simulink model "Simulink_PMSM"  (R2022b)
settings: Solver=VariableStepAuto  StartTime=0.0  StopTime=3.5  FixedStep=Ts  MaxStep=1e-5  RelTol=1e-3  AbsTol=1e-3  EnableMultiTasking=on
PreLoadFcn:
  | % PMSM parameters
  | PM = 0.005237624506507; % Permanent magnet flux linkage
  | Ld = 0.00105;  % d-axis inductance
  | Lq = 0.00105;  % q-axis inductance
  | L0 = 0.00105;  % 0-axis inductance
  | Rs = 0.75; % Stator resistance
  | N = 4; % Number of pole pairs
  | J = 2.4018552467e-06; % Moment of inertia
  | B = 1.160371049300000e-05; % Damping
  | 
  | % Operating and derived limits
  | Trated = 0.056566344670276 %Par nominal
values from neighbouring files (symbols this model uses):
  fsw = 1e3    (= 1000)    [Variables_simulink_PMSM.m]
  Kiid = 2    [Variables_simulink_PMSM.m]
  Kiiq = Kpiq    (= 1)    [Variables_simulink_PMSM.m]
  Kivel = 3    [Variables_simulink_PMSM.m]
  Kpid = 1    [Variables_simulink_PMSM.m]
  Kpiq = Kpid    (= 1)    [Variables_simulink_PMSM.m]
  Kpvel = 6    [Variables_simulink_PMSM.m]
  Refvel = 300    [Variables_simulink_PMSM.m]
  Tcurr = 1e-4    (= 0.0001)    [Variables_simulink_PMSM.m]
  Ts = 1e-6    (= 1e-06)    [Variables_simulink_PMSM.m]
  Tspeed = 2e-4    (= 0.0002)    [Variables_simulink_PMSM.m]
  Tsw = 5e-7    (= 5e-07)    [Variables_simulink_PMSM.m]
  Vbat = 48    [Variables_simulink_PMSM.m]
libraries: slpidlib x3, eePwmGenerator x3, eeTransforms x2, simulink x1, eePwmGeneratorTwoLevel x1, autolibpmsmexterior x1
Description:
  | Three-Phase PMSM Drive
settings Model: Creator=The MathWorks, Inc.  LastModifiedBy=emate
settings SolverCC: AutoScaleAbsTol=off  MaxConsecutiveMinStep=2  ZeroCrossAlgorithm=Adaptive  AlgebraicLoopSolver=TrustRegion  MaxZcPerStep=1
settings DataIOCC: LimitDataPoints=on  MaxDataPoints=690000  SaveFormat=Array  ReturnWorkspaceOutputs=off  SignalLoggingName=logsout_ee_pmsm_drive
settings OptimizationCC: LifeSpan=inf
settings DebuggingCC: MaxConsecutiveZCsMsg=none  IgnoredZcDiagnostic=none  UnconnectedInputMsg=warning  UnconnectedOutputMsg=warning  UnconnectedLineMsg=warning  AllowSymbolicDim=off  PregeneratedLibrarySubsystemCodeDiagnostic=none  SFUnexpectedBacktrackingDiag=warning  SFNoUnconditionalDefaultTransitionDiag=warning  SFExecutionAtInitializationDiag=none  SFMachineParentedDataDiag=warning  ArithmeticOperatorsInVariantConditions=warning
settings HardwareCC: ProdBitPerPointer=32  ProdBitPerSizeT=32  ProdBitPerPtrDiffT=32  ProdLargestAtomicFloat=None  ProdIntDivRoundTo=Undefined  ProdEndianess=Unspecified  ProdWordSize=32  ProdHWDeviceType=32-bit Generic
settings ModelReferenceCC: EnableRefExpFcnMdlSchedulingChecks=on  PropagateSignalLabelsOutOfModel=off
settings SFSimCC: SimUseLocalCustomCode=off
settings RTWCC: RTWUseLocalCustomCode=off  DLArmComputeVersion=19.05
settings CodeAppCC: StateflowObjectComments=on
settings GRTTargetCC: TargetLangStandard=C89/C90 (ANSI)
settings ConfigComp: CovMetricSettings=dw  CovSaveCumulativeToWorkspaceVar=on  CovSaveSingleToWorkspaceVar=on  CovExternalEMLEnable=off  CovSFcnEnable=off
settings SimscapeCC: SimscapeLogType=all  SimscapeLogSimulationStatistics=on  SimscapeLogName=simlog_ee_pmsm_drive  SimscapeLogDataHistory=690000

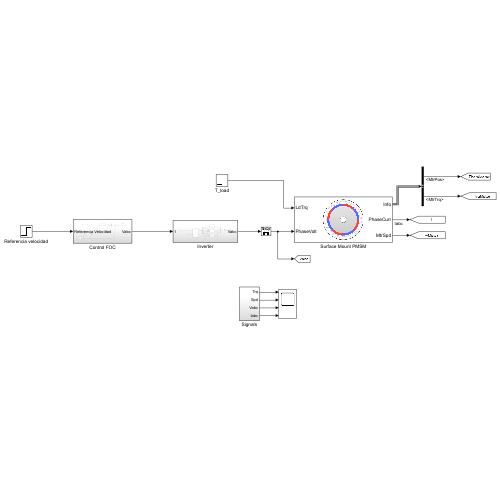
[thumbnail: Simulink's stored preview of the top-level diagram]
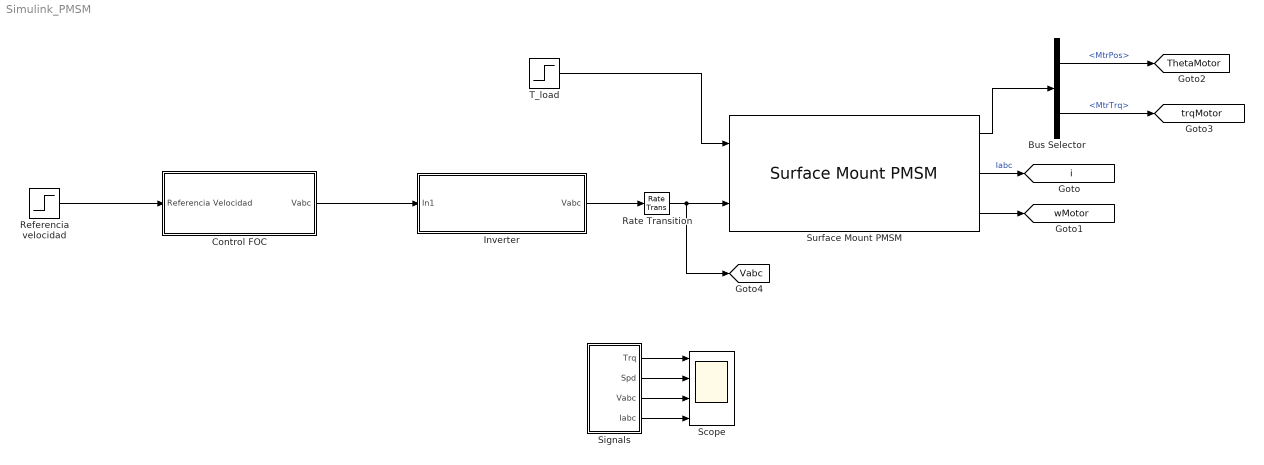
== system Simulink_PMSM ==
  Bus Selector : BusSelector  OutputSignals=MtrPos,MtrTrq
  Control FOC : Subsystem
  Inverter : Subsystem
  Rate Transition : RateTransition  Deterministic=off  OutPortSampleTime=Tsw
  Referencia velocidad : Step  Time=0.5  After=Refvel  SampleTime=Tspeed
  Scope : Scope  NumInputPorts=4
  "Signals " : Subsystem
  Surface Mount PMSM : autolibpmsmexterior/Surface Mount PMSM  port_config=Torque  sim_type=Discrete  Ts=Ts  P=N  Rs=Rs  Ldq_=Ld  KConstText=Permanent flux linkage constant (lambda_pm):  lambda_pm=PM  Ke=159.9771  Kt=1.323  mechanical=[J*1e4, B*5, 0]  idq0=[0 0]  theta_init=0  omega_init=0  KConst=PM  lambda_pm_calc=PM  RefBlkName='autolibpmsmexterior/Surface Mount PMSM'  aMode=5  Ldq="[0.0006      0.0006]"
  T_load : Step  Time=2  After=0.75*Trated  SampleTime=Ts
  tag scope: ThetaMotor=global, Vabc=global, i=global, trqMotor=global, wMotor=global
  wires:
  "Signals "/2(Spd) -> Scope/2
  "Signals "/1(Trq) -> Scope/1
  "Signals "/3(Vabc) -> Scope/3
  "Signals "/4(Iabc) -> Scope/4
  Referencia velocidad/1 -> Control FOC/1(Referencia Velocidad)
  Control FOC/1(Vabc) -> Inverter/1(In1)
  Rate Transition/1 -> [Vabc], Surface Mount PMSM/2
  T_load/1 -> Surface Mount PMSM/1
  Surface Mount PMSM/3 -> [wMotor]
  Surface Mount PMSM/2 -> [i]  "Iabc"
  Surface Mount PMSM/1 -> Bus Selector/1
  Bus Selector/1 -> [ThetaMotor]  "<MtrPos>"
  Bus Selector/2 -> [trqMotor]  "<MtrTrq>"
  Inverter/1(Vabc) -> Rate Transition/1

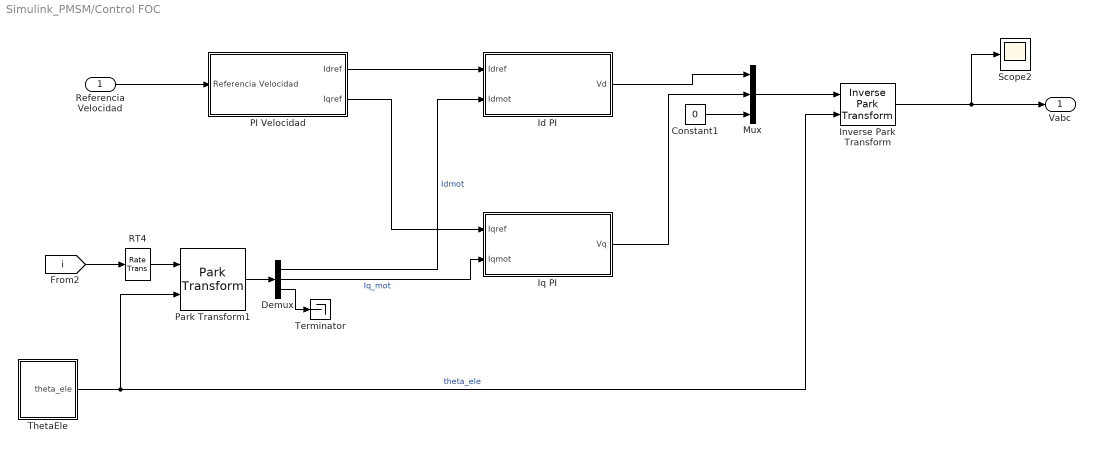
== system Simulink_PMSM/Control FOC ==
  Referencia Velocidad : Inport
  Constant1 : Constant  Value=0  SampleTime=Tcurr
  Demux : Demux  Outputs=3
  Id PI : Subsystem
  Inverse Park Transform : eeTransforms/Inverse Park Transform  AxisAlignment=D-axis  PowerInvariant=off
  Iq PI : Subsystem
  Mux : Mux  Inputs=3
  PI Velocidad : Subsystem
  Park Transform1 : eeTransforms/Park Transform  AxisAlignment=D-axis  PowerInvariant=off
      settings: LibrarySourceBlock=|
      | ee_sl_lib/Mathematical
      | Transforms/Park Transform
  RT4 : RateTransition  InitialCondition=[0,0,0]  OutPortSampleTime=Tspeed
  Scope2 : Scope
  Terminator : Terminator
  ThetaEle : Subsystem
  Vabc : Outport
  wires:
  PI Velocidad/1(Idref) -> Id PI/1(Idref)
  Constant1/1 -> Mux/3
  PI Velocidad/2(Iqref) -> Iq PI/1(Iqref)
  [i] -> RT4/1
  Demux/2 -> Iq PI/2(Iqmot)  "Iq_mot"
  ThetaEle/1(theta_ele) -> Inverse Park Transform/2, Park Transform1/2  "theta_ele"
  Iq PI/1(Vq) -> Mux/2
  Id PI/1(Vd) -> Mux/1
  Inverse Park Transform/1 -> Scope2/1, Vabc/1
  Demux/3 -> Terminator/1
  Demux/1 -> Id PI/2(Idmot)  "Idmot"
  Park Transform1/1 -> Demux/1
  RT4/1 -> Park Transform1/1
  Mux/1 -> Inverse Park Transform/1
  Referencia Velocidad/1 -> PI Velocidad/1(Referencia Velocidad)

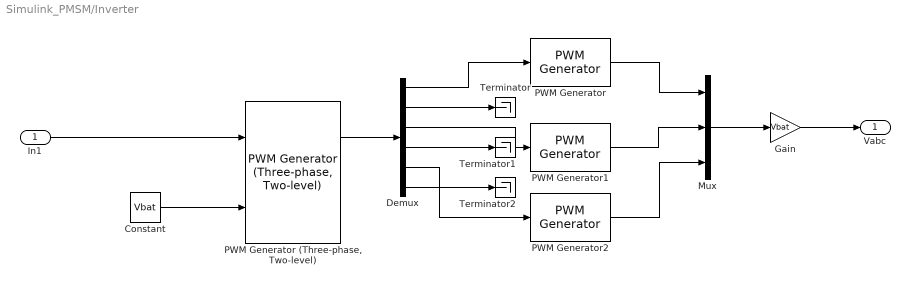
== system Simulink_PMSM/Inverter ==
  In1 : Inport
  Constant : Constant  Value=Vbat
  Demux : Demux  Outputs=6
  Gain : Gain  Gain=Vbat
  Mux : Mux  Inputs=3
  PWM Generator : eePwmGenerator/PWM Generator  CarrCount=Up  Tper=1/fsw  Tdelay=0  Ts=Tsw
  "PWM Generator (Three-phase, Two-level)" : eePwmGeneratorTwoLevel/PWM Generator (Three-phase, Two-level)  PWMMode=Continuous PWM (CPWM)  CPWMMode=SPWM: sinusoidal PWM  DPWMMode=60 DPWM: 60 degree discontinuous PWM  fsw=fsw  Ts=Tsw
      settings: LibrarySourceBlock=|
      | eePmsmFieldOrientedControl/PMSM Field-Oriented
      | Control/PWM/PWM Generator
      | (Three-phase, Two-level)
  PWM Generator1 : eePwmGenerator/PWM Generator  CarrCount=Up  Tper=1/fsw  Tdelay=0  Ts=Tsw
  PWM Generator2 : eePwmGenerator/PWM Generator  CarrCount=Up  Tper=1/fsw  Tdelay=0  Ts=Tsw
  Terminator : Terminator
  Terminator1 : Terminator
  Terminator2 : Terminator
  Vabc : Outport  VectorParamsAs1DForOutWhenUnconnected=off
  wires:
  In1/1 -> "PWM Generator (Three-phase, Two-level)"/1
  Mux/1 -> Gain/1
  Constant/1 -> "PWM Generator (Three-phase, Two-level)"/2
  "PWM Generator (Three-phase, Two-level)"/1 -> Demux/1
  Demux/2 -> Terminator/1
  Demux/4 -> Terminator1/1
  Demux/6 -> Terminator2/1
  PWM Generator/1 -> Mux/1
  Demux/1 -> PWM Generator/1
  Demux/3 -> PWM Generator1/1
  Demux/5 -> PWM Generator2/1
  PWM Generator1/1 -> Mux/2
  PWM Generator2/1 -> Mux/3
  Gain/1 -> Vabc/1

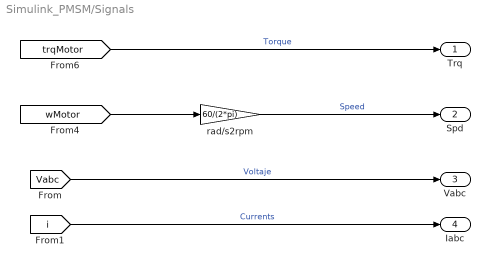
== system Simulink_PMSM/Signals  ==
  rad/s2rpm : Gain  Gain=60/(2*pi)
  Trq : Outport  VectorParamsAs1DForOutWhenUnconnected=off
  Spd : Outport  Port=2  VectorParamsAs1DForOutWhenUnconnected=off
  Vabc : Outport  Port=3  VectorParamsAs1DForOutWhenUnconnected=off
  Iabc : Outport  Port=4  VectorParamsAs1DForOutWhenUnconnected=off
  wires:
  [wMotor] -> rad/s2rpm/1
  [trqMotor] -> Trq/1  "Torque"
  [Vabc] -> Vabc/1  "Voltaje"
  rad/s2rpm/1 -> Spd/1  "Speed"
  [i] -> Iabc/1  "Currents"

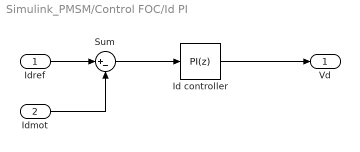
== system Simulink_PMSM/Control FOC/Id PI ==
  Idref : Inport
  Idmot : Inport  Port=2
  Id controller : slpidlib/PID Controller  Controller=PI  Form=Parallel  TimeDomain=Discrete-time  UseExternalTs=off  SampleTime=Tcurr  IntegratorMethod=Forward Euler  FilterMethod=Forward Euler  ControllerParametersSource=internal  P=Kpid  I=Kiid  UseKiTs=off  D=0  N=100  UseFilter=on  TunerSelectOption=Transfer Function Based (PID Tuner App)  InitialConditionSource=internal  InitialConditionForIntegrator=0  InitialConditionForFilter=0  DifferentiatorICPrevScaledInput=0  ExternalReset=none  TrackingMode=off  Kt=1  LimitOutput=on  SatLimitsSource=internal  UpperSaturationLimit=inf  LowerSaturationLimit=-inf  LinearizeAsGain=on  AntiWindupMode=clamping  Kb=1000  LimitIntegrator=off  UpperIntegratorSaturationLimit=inf  LowerIntegratorSaturationLimit=-inf  POutMin=[]  POutMax=[]  IOutMin=[]  IOutMax=[]  DOutMin=[]  DOutMax=[]  NOutMin=[]  NOutMax=[]  SumOutMin=[]  SumOutMax=[]  SaturationOutMin=[]  SaturationOutMax=[]  PParamMin=[]  PParamMax=[]  IParamMin=[]  IParamMax=[]  DParamMin=[]  DParamMax=[]  NParamMin=[]  NParamMax=[]  KbParamMin=[]  KbParamMax=[]  KtParamMin=[]  KtParamMax=[]  KbOutMin=[]  KbOutMax=[]  KtOutMin=[]  KtOutMax=[]  IntegratorOutMin=[]  IntegratorOutMax=[]  FilterOutMin=[]  FilterOutMax=[]  SumI1OutMin=[]  SumI1OutMax=[]  SumI2OutMin=[]  SumI2OutMax=[]  SumI3OutMin=[]  SumI3OutMax=[]  SumI4OutMin=[]  SumI4OutMax=[]  SumDOutMin=[]  SumDOutMax=[]  DifferentiatorOutMin=[]  DifferentiatorOutMax=[]  FilterDiffOutCoefMin=[]  FilterDiffOutCoefMax=[]  ReciprocalOutMin=[]  ReciprocalOutMax=[]  SumDenOutMin=[]  SumDenOutMax=[]  SumNumOutMin=[]  SumNumOutMax=[]  DivideOutMin=[]  DivideOutMax=[]  UdiffTsProdOutMin=[]  UdiffTsProdOutMax=[]  NTsProdOutMin=[]  NTsProdOutMax=[]  UintegralTsProdOutMin=[]  UintegralTsProdOutMax=[]  UngainTsProdOutMin=[]  UngainTsProdOutMax=[]  ClampingZeroOutDataTypeStr=Inherit: Inherit via back propagation  ClampingZeroOutMin=[]  ClampingZeroOutMax=[]  FilterDenConstantOutDataTypeStr=Inherit: Inherit via back propagation  FilterDenConstantOutMin=[]  FilterDenConstantOutMax=[]  PCopyOutDataTypeStr=Inherit: Inherit via back propagation  PCopyOutMin=[]  PCopyOutMax=[]  NCopyOutDataTypeStr=Inherit: Inherit via back propagation  NCopyOutMin=[]  NCopyOutMax=[]  IntegratorContinuousStateAttributes=''  IntegratorStateMustResolveToSignalObject=off  IntegratorRTWStateStorageClass=Auto  FilterContinuousStateAttributes=''  FilterStateMustResolveToSignalObject=off  FilterRTWStateStorageClass=Auto  ParallelPVariant=InternalParameters  IdealPVariant=Disabled  IVariant=InternalParameters  DVariant=Disabled  IntegratorVariant=Discrete  SatVariant=Enabled  AWVariant=DiscClampingParallel  PCopyVariant=Disabled  TRVariant=Disabled  FdbkBlocksVariant=Forward  IdealPFdbkVariant=Disabled  SatFdbkVariant=Disabled  DerivativeFilterVariant=Disabled  NVariant=Disabled  NCopyVariant=Disabled_SignalSpec  FilterICVariant=Disabled  IntegratorICVariant=InternalICs  ExternalResetVariant=Disabled  TRSumVariant=Passthrough  SumFdbkVariant=Disabled  SumVariant=Sum_PI  TsampFilterVariant=InternalTs  TsampNgainVariant=Passthrough  TsampIntegralVariant=Passthrough  ExternalSaturationOutDataTypeStr=Inherit: Same as second input
  Sum : Sum  Inputs=|+-
  Vd : Outport
  wires:
  Idmot/1 -> Sum/2
  Idref/1 -> Sum/1
  Id controller/1 -> Vd/1
  Sum/1 -> Id controller/1

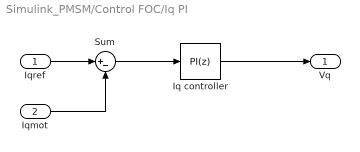
== system Simulink_PMSM/Control FOC/Iq PI ==
  Iqref : Inport
  Iqmot : Inport  Port=2
  Iq controller : slpidlib/PID Controller  Controller=PI  Form=Parallel  TimeDomain=Discrete-time  UseExternalTs=off  SampleTime=Tcurr  IntegratorMethod=Forward Euler  FilterMethod=Forward Euler  ControllerParametersSource=internal  P=Kpiq  I=Kiiq  UseKiTs=off  D=0  N=100  UseFilter=on  TunerSelectOption=Transfer Function Based (PID Tuner App)  InitialConditionSource=internal  InitialConditionForIntegrator=0  InitialConditionForFilter=0  DifferentiatorICPrevScaledInput=0  ExternalReset=none  TrackingMode=off  Kt=1  LimitOutput=on  SatLimitsSource=internal  UpperSaturationLimit=inf  LowerSaturationLimit=-inf  LinearizeAsGain=on  AntiWindupMode=clamping  Kb=1000  LimitIntegrator=off  UpperIntegratorSaturationLimit=inf  LowerIntegratorSaturationLimit=-inf  POutMin=[]  POutMax=[]  IOutMin=[]  IOutMax=[]  DOutMin=[]  DOutMax=[]  NOutMin=[]  NOutMax=[]  SumOutMin=[]  SumOutMax=[]  SaturationOutMin=[]  SaturationOutMax=[]  PParamMin=[]  PParamMax=[]  IParamMin=[]  IParamMax=[]  DParamMin=[]  DParamMax=[]  NParamMin=[]  NParamMax=[]  KbParamMin=[]  KbParamMax=[]  KtParamMin=[]  KtParamMax=[]  KbOutMin=[]  KbOutMax=[]  KtOutMin=[]  KtOutMax=[]  IntegratorOutMin=[]  IntegratorOutMax=[]  FilterOutMin=[]  FilterOutMax=[]  SumI1OutMin=[]  SumI1OutMax=[]  SumI2OutMin=[]  SumI2OutMax=[]  SumI3OutMin=[]  SumI3OutMax=[]  SumI4OutMin=[]  SumI4OutMax=[]  SumDOutMin=[]  SumDOutMax=[]  DifferentiatorOutMin=[]  DifferentiatorOutMax=[]  FilterDiffOutCoefMin=[]  FilterDiffOutCoefMax=[]  ReciprocalOutMin=[]  ReciprocalOutMax=[]  SumDenOutMin=[]  SumDenOutMax=[]  SumNumOutMin=[]  SumNumOutMax=[]  DivideOutMin=[]  DivideOutMax=[]  UdiffTsProdOutMin=[]  UdiffTsProdOutMax=[]  NTsProdOutMin=[]  NTsProdOutMax=[]  UintegralTsProdOutMin=[]  UintegralTsProdOutMax=[]  UngainTsProdOutMin=[]  UngainTsProdOutMax=[]  ClampingZeroOutDataTypeStr=Inherit: Inherit via back propagation  ClampingZeroOutMin=[]  ClampingZeroOutMax=[]  FilterDenConstantOutDataTypeStr=Inherit: Inherit via back propagation  FilterDenConstantOutMin=[]  FilterDenConstantOutMax=[]  PCopyOutDataTypeStr=Inherit: Inherit via back propagation  PCopyOutMin=[]  PCopyOutMax=[]  NCopyOutDataTypeStr=Inherit: Inherit via back propagation  NCopyOutMin=[]  NCopyOutMax=[]  IntegratorContinuousStateAttributes=''  IntegratorStateMustResolveToSignalObject=off  IntegratorRTWStateStorageClass=Auto  FilterContinuousStateAttributes=''  FilterStateMustResolveToSignalObject=off  FilterRTWStateStorageClass=Auto  ParallelPVariant=InternalParameters  IdealPVariant=Disabled  IVariant=InternalParameters  DVariant=Disabled  IntegratorVariant=Discrete  SatVariant=Enabled  AWVariant=DiscClampingParallel  PCopyVariant=Disabled  TRVariant=Disabled  FdbkBlocksVariant=Forward  IdealPFdbkVariant=Disabled  SatFdbkVariant=Disabled  DerivativeFilterVariant=Disabled  NVariant=Disabled  NCopyVariant=Disabled_SignalSpec  FilterICVariant=Disabled  IntegratorICVariant=InternalICs  ExternalResetVariant=Disabled  TRSumVariant=Passthrough  SumFdbkVariant=Disabled  SumVariant=Sum_PI  TsampFilterVariant=InternalTs  TsampNgainVariant=Passthrough  TsampIntegralVariant=Passthrough  ExternalSaturationOutDataTypeStr=Inherit: Same as second input
  Sum : Sum  Inputs=|+-
  Vq : Outport
  wires:
  Iq controller/1 -> Vq/1
  Sum/1 -> Iq controller/1
  Iqref/1 -> Sum/1
  Iqmot/1 -> Sum/2

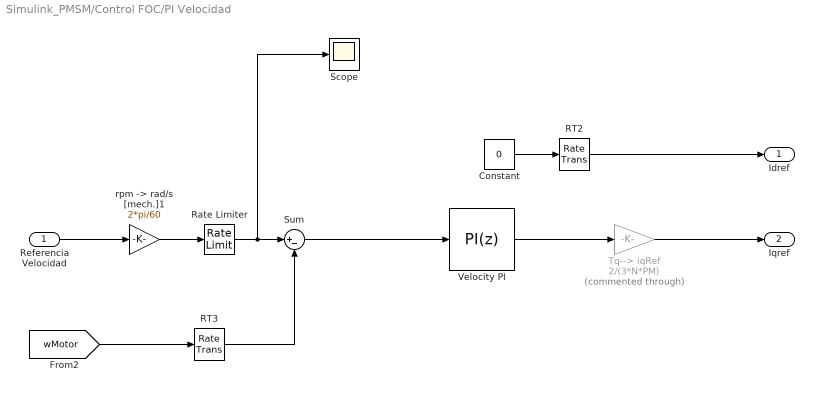
== system Simulink_PMSM/Control FOC/PI Velocidad ==
  Referencia Velocidad : Inport
  Constant : Constant  Value=0
  RT2 : RateTransition  OutPortSampleTime=Tspeed
  RT3 : RateTransition  OutPortSampleTime=Tspeed
  Rate Limiter : RateLimiter  RisingSlewLimit=50  FallingSlewLimit=-50  SampleTimeMode=inherited
  Scope : Scope
  Sum : Sum  Inputs=|+-
  Tq--> iqRef : Gain  Commented=through  Gain=2/(3*N*PM)
  Velocity PI : slpidlib/PID Controller  Controller=PI  Form=Parallel  TimeDomain=Discrete-time  UseExternalTs=off  SampleTime=Tspeed  IntegratorMethod=Trapezoidal  FilterMethod=Forward Euler  ControllerParametersSource=internal  P=Kpvel  I=Kivel  UseKiTs=off  D=0  N=100  UseFilter=on  TunerSelectOption=Transfer Function Based (PID Tuner App)  InitialConditionSource=internal  InitialConditionForIntegrator=0  InitialConditionForFilter=0  DifferentiatorICPrevScaledInput=0  ExternalReset=none  TrackingMode=off  Kt=1  LimitOutput=on  SatLimitsSource=internal  UpperSaturationLimit=inf  LowerSaturationLimit=-inf  LinearizeAsGain=on  AntiWindupMode=clamping  Kb=1000  LimitIntegrator=off  UpperIntegratorSaturationLimit=inf  LowerIntegratorSaturationLimit=-inf  POutMin=[]  POutMax=[]  IOutMin=[]  IOutMax=[]  DOutMin=[]  DOutMax=[]  NOutMin=[]  NOutMax=[]  SumOutMin=[]  SumOutMax=[]  SaturationOutMin=[]  SaturationOutMax=[]  PParamMin=[]  PParamMax=[]  IParamMin=[]  IParamMax=[]  DParamMin=[]  DParamMax=[]  NParamMin=[]  NParamMax=[]  KbParamMin=[]  KbParamMax=[]  KtParamMin=[]  KtParamMax=[]  KbOutMin=[]  KbOutMax=[]  KtOutMin=[]  KtOutMax=[]  IntegratorOutMin=[]  IntegratorOutMax=[]  FilterOutMin=[]  FilterOutMax=[]  SumI1OutMin=[]  SumI1OutMax=[]  SumI2OutMin=[]  SumI2OutMax=[]  SumI3OutMin=[]  SumI3OutMax=[]  SumI4OutMin=[]  SumI4OutMax=[]  SumDOutMin=[]  SumDOutMax=[]  DifferentiatorOutMin=[]  DifferentiatorOutMax=[]  FilterDiffOutCoefMin=[]  FilterDiffOutCoefMax=[]  ReciprocalOutMin=[]  ReciprocalOutMax=[]  SumDenOutMin=[]  SumDenOutMax=[]  SumNumOutMin=[]  SumNumOutMax=[]  DivideOutMin=[]  DivideOutMax=[]  UdiffTsProdOutMin=[]  UdiffTsProdOutMax=[]  NTsProdOutMin=[]  NTsProdOutMax=[]  UintegralTsProdOutMin=[]  UintegralTsProdOutMax=[]  UngainTsProdOutMin=[]  UngainTsProdOutMax=[]  ClampingZeroOutDataTypeStr=Inherit: Inherit via back propagation  ClampingZeroOutMin=[]  ClampingZeroOutMax=[]  FilterDenConstantOutDataTypeStr=Inherit: Inherit via back propagation  FilterDenConstantOutMin=[]  FilterDenConstantOutMax=[]  PCopyOutDataTypeStr=Inherit: Inherit via back propagation  PCopyOutMin=[]  PCopyOutMax=[]  NCopyOutDataTypeStr=Inherit: Inherit via back propagation  NCopyOutMin=[]  NCopyOutMax=[]  IntegratorContinuousStateAttributes=''  IntegratorStateMustResolveToSignalObject=off  IntegratorRTWStateStorageClass=Auto  FilterContinuousStateAttributes=''  FilterStateMustResolveToSignalObject=off  FilterRTWStateStorageClass=Auto  ParallelPVariant=InternalParameters  IdealPVariant=Disabled  IVariant=InternalParameters  DVariant=Disabled  IntegratorVariant=Discrete  SatVariant=Enabled  AWVariant=DiscClampingParallel  PCopyVariant=Disabled  TRVariant=Disabled  FdbkBlocksVariant=Feedback  IdealPFdbkVariant=Passthrough  SatFdbkVariant=Passthrough  DerivativeFilterVariant=Disabled  NVariant=Disabled  NCopyVariant=Disabled_SignalSpec  FilterICVariant=Disabled  IntegratorICVariant=InternalICs  ExternalResetVariant=Disabled  TRSumVariant=Passthrough  SumFdbkVariant=Enabled  SumVariant=Sum_PI  TsampFilterVariant=InternalTs  TsampNgainVariant=Passthrough  TsampIntegralVariant=Passthrough  ExternalSaturationOutDataTypeStr=Inherit: Same as second input
  "rpm -> rad/s [mech.]1" : Gain  Gain=2*pi/60
  Idref : Outport
  Iqref : Outport  Port=2
  wires:
  Referencia Velocidad/1 -> "rpm -> rad/s [mech.]1"/1
  Sum/1 -> Velocity PI/1
  Constant/1 -> RT2/1
  RT2/1 -> Idref/1
  Tq--> iqRef/1 -> Iqref/1
  Velocity PI/1 -> Tq--> iqRef/1
  [wMotor] -> RT3/1
  "rpm -> rad/s [mech.]1"/1 -> Rate Limiter/1
  Rate Limiter/1 -> Scope/1, Sum/1
  RT3/1 -> Sum/2

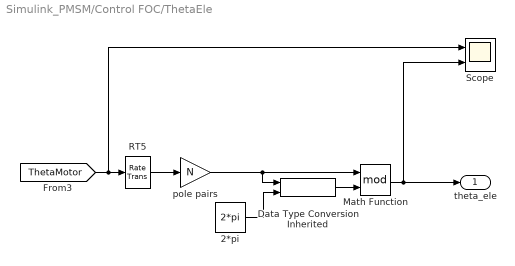
== system Simulink_PMSM/Control FOC/ThetaEle ==
  2*pi : Constant  Value=2*pi  OutDataTypeStr=Inherit: Inherit via back propagation  SampleTime=2e-4
  Data Type Conversion Inherited : simulink/Signal Attributes/Data Type Conversion Inherited  ConvertRealWorld=Real World Value  DoSatur=off
  Math Function : Math  Operator=mod  SignedPower=on
  RT5 : RateTransition  OutPortSampleTime=Tspeed
  Scope : Scope  NumInputPorts=2
  "pole pairs " : Gain  Gain=N
  theta_ele : Outport  VectorParamsAs1DForOutWhenUnconnected=off
  wires:
  [ThetaMotor] -> Scope/1, RT5/1
  Math Function/1 -> Scope/2, theta_ele/1
  RT5/1 -> "pole pairs "/1
  2*pi/1 -> Data Type Conversion Inherited/2
  "pole pairs "/1 -> Data Type Conversion Inherited/1, Math Function/1
  Data Type Conversion Inherited/1 -> Math Function/2
